simulink model "smc_diff_with_plant"  (R2024b)
settings: Solver=ode1  StartTime=0.0  StopTime=30  FixedStep=1e-5  RelTol=1e-3
libraries: simulink x1
settings Model: Creator=user  LastModifiedBy=user

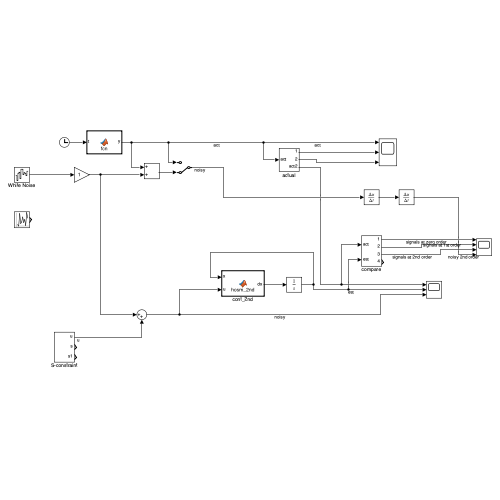
[thumbnail: Simulink's stored preview of the top-level diagram]
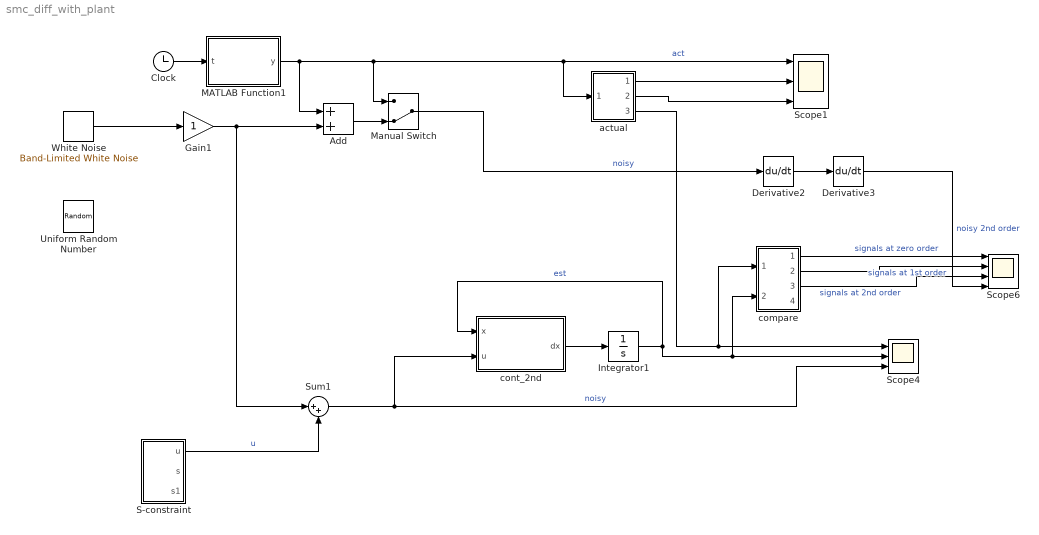
== system smc_diff_with_plant ==
  Add : Sum
  Clock : Clock
  Derivative2 : Derivative
  Derivative3 : Derivative
  Gain1 : Gain
  Integrator1 : Integrator
  MATLAB Function1 : MATLAB Function  TreatAsAtomicUnit=on
  Manual Switch : ManualSwitch  CurrentSetting=0
  S-constraint : Subsystem
  Scope1 : Scope  NumInputPorts=3
  Scope4 : Scope  NumInputPorts=3
  Scope6 : Scope  NumInputPorts=4
  Sum1 : Sum  Inputs=|++
  Uniform Random Number : UniformRandomNumber  Minimum=-1e-3  Maximum=1e-3  SampleTime=0.001
  White Noise : simulink/Sources/Band-Limited White Noise  Cov=1e-8*1  Ts=0.001  seed=[23341]
  actual : Subsystem
  compare : Subsystem
  cont_2nd : MATLAB Function  TreatAsAtomicUnit=on
  wires:
  Clock/1 -> MATLAB Function1/1(t)
  cont_2nd/1(dx) -> Integrator1/1
  Integrator1/1 -> cont_2nd/1(x), Scope4/2, compare/2(est)  "est"
  Sum1/1 -> Scope4/3, cont_2nd/2(u)  "noisy"
  Add/1 -> Manual Switch/2
  MATLAB Function1/1(y) -> Scope1/1, actual/1(act), Manual Switch/1, Add/1  "act"
  Manual Switch/1 -> Derivative2/1  "noisy"
  S-constraint/1(u) -> Sum1/2  "u"
  compare/1(Out1) -> Scope6/1  "signals at zero order"
  compare/2(Out2) -> Scope6/2  "signals at 1st order"
  compare/3(Out3) -> Scope6/3  "signals at 2nd order"
  Derivative2/1 -> Derivative3/1
  Derivative3/1 -> Scope6/4  "noisy 2nd order"
  Gain1/1 -> Sum1/1, Add/2
  White Noise/1 -> Gain1/1
  actual/3(act2) -> Scope4/1, compare/1(act)
  actual/1(Out1) -> Scope1/2
  actual/2(Out2) -> Scope1/3

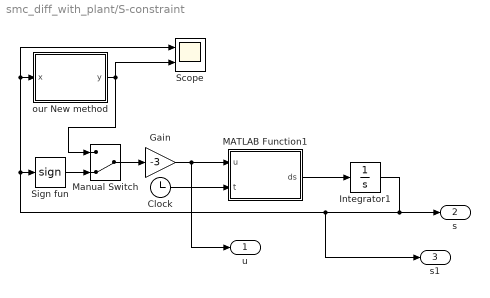
== system smc_diff_with_plant/S-constraint ==
  Clock : Clock
  Gain : Gain  Gain=-3
  Integrator1 : Integrator  InitialCondition=5
  MATLAB Function1 : MATLAB Function  TreatAsAtomicUnit=on
  Manual Switch : ManualSwitch  CurrentSetting=0
  Scope : Scope  NumInputPorts=2
  Sign fun : Signum
  "our New method " : MATLAB Function  TreatAsAtomicUnit=on
  u : Outport
  s : Outport  Port=2
  s1 : Outport  Port=3
  wires:
  MATLAB Function1/1(ds) -> Integrator1/1
  Clock/1 -> MATLAB Function1/2(t)
  Gain/1 -> MATLAB Function1/1(u), u/1
  "our New method "/1(y) -> Manual Switch/1, Scope/2
  Sign fun/1 -> Manual Switch/2
  Manual Switch/1 -> Gain/1
  Integrator1/1 -> s1/1, Sign fun/1, Scope/1, "our New method "/1(x), s/1

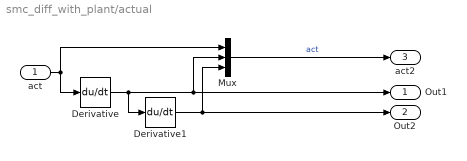
== system smc_diff_with_plant/actual ==
  act : Inport
  Derivative : Derivative
  Derivative1 : Derivative
  Mux : Mux  Inputs=3
  Out1 : Outport
  Out2 : Outport  Port=2
  act2 : Outport  Port=3
  wires:
  Mux/1 -> act2/1  "act"
  act/1 -> Derivative/1, Mux/1
  Derivative/1 -> Out1/1, Mux/2, Derivative1/1
  Derivative1/1 -> Out2/1, Mux/3

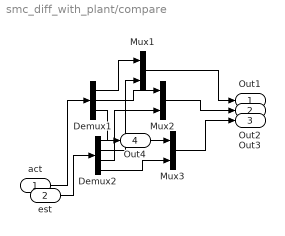
== system smc_diff_with_plant/compare ==
  act : Inport
  est : Inport  Port=2
  Demux1 : Demux  Outputs=3
  Demux2 : Demux  Outputs=[2 1 1 1]
  Mux1 : Mux  Inputs=2
  Mux2 : Mux  Inputs=2
  Mux3 : Mux  Inputs=2
  Out1 : Outport
  Out2 : Outport  Port=2
  Out3 : Outport  Port=3
  Out4 : Outport  Port=4
  wires:
  act/1 -> Demux1/1
  Demux1/2 -> Mux2/1
  Mux3/1 -> Out3/1
  Demux2/1 -> Out4/1
  Demux1/1 -> Mux1/1
  Demux2/4 -> Mux3/2
  Mux1/1 -> Out1/1
  Demux2/2 -> Mux1/2
  est/1 -> Demux2/1
  Mux2/1 -> Out2/1
  Demux1/3 -> Mux3/1
  Demux2/3 -> Mux2/2

== matlab function smc_diff_with_plant/S-constraint/MATLAB Function1 ==
  data: u input; ds output; t input
function ds = fcn(u, t)
    %ds = cos(t) + (2 + sin(3*t))*u;
    ds = (1+exp(-2*t))*sin(2*t) + (5 + cos(t))*u;
end

== matlab function smc_diff_with_plant/MATLAB Function1 ==
  data: t input; y output
function y = fcn(t)

%y = -cos(t)/(2+sin(3*t));
y = -(1+exp(-2*t))*sin(2*t)/(5+cos(t));

== matlab function smc_diff_with_plant/S-constraint/our New method  ==
  data: x input; y output
% function y = bisigmoid(x)
%     k = 1e4; c = 1;
%     y = tanh(k * x);
% end

function y = alevantbook(x)

  y = x/(abs(x)+1e-8);

end

== matlab function smc_diff_with_plant/cont_2nd ==
  data: x input; u input; dx output
function dx = hosm_2nd(x, u)

%
dx = zeros(5, 1);
L = 35; % Lipschetz boundary
gamma = 1;
lambda = [1.1 3.06, 4.16 3];

z_m2 = x(1);   % z_{-2}
z_m1 = x(2);   % z_{-1}
z0   = x(3);   % z_0, estimate of u_eq
z1   = x(4);   % z_1, estimate of u_eq derivative
z2   = x(5);   % z_2, estimate of u_eq second derivative

% Extract lambda parameters:
lambda0 = lambda(1);
lambda1 = lambda(2);
lambda2 = lambda(3);
lambda3 = lambda(4);

% error
e = z_m1 - z_m2;

% Define the fractional power function:
% fpower(w, alpha) = |w|^alpha * sign(w)
fpower = @(w, alpha) (abs(w)^alpha) * sign(w);


dz_m2 = u - gamma * z_m2;

dz_m1 = -lambda3 * L^(1/4) * fpower(e, 3/4) + z0 - gamma * z_m2;
dz0   = -lambda2 * L^(2/4) * fpower(e, 2/4) + z1;
dz1   = -lambda1 * L^(3/4) * fpower(e, 1/4) + z2;
dz2   = -lambda0 * L * sign(e);

%-----------------------------------------------------------------------
% Assemble the state derivative vector:
dx = [dz_m2; dz_m1; dz0; dz1; dz2];

end
